simulink model "Three_phase_twelve_pulse_wave"  (R2025a)
settings: Solver=VariableStepAuto  StartTime=0.0  StopTime=0.06  MaxStep=1e-4  RelTol=1e-3
undefined symbols (not defined in the file): D1, Delta, lagging, pulse
libraries: spsUniversalBridgeLib x2, spsGroundLib x1, spsMultimeterLib x1, spsPLL3phLib x1, spsPulseGeneratorThyristor12PulseLib x1, spsSeriesRLCBranchLib x1, spsThreePhaseProgrammableVoltageSourceLib x1, spsThreePhaseVIMeasurementLib x1, spsThreePhaseTransformerThreeWindingsLib x1, sps_lib x1
settings Model: Creator=wz  LastModifiedBy=wz

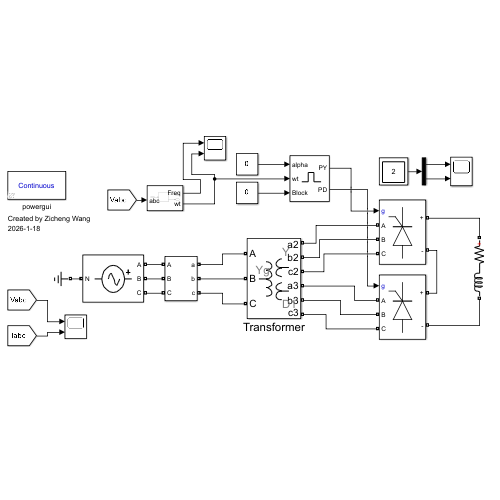
[thumbnail: Simulink's stored preview of the top-level diagram]
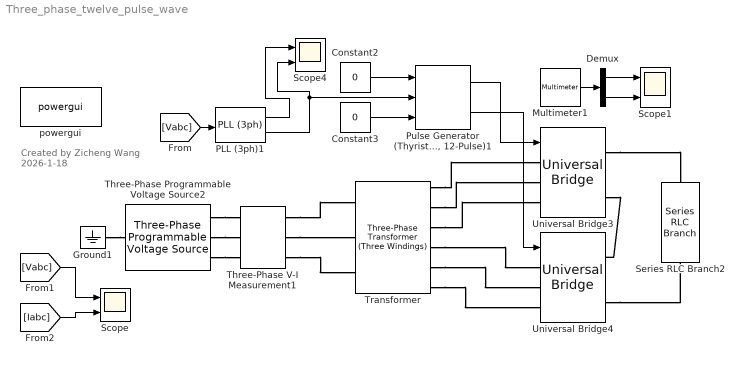
== system Three_phase_twelve_pulse_wave ==
  note: Created by Zicheng Wang
      | 2026-1-18
  Constant2 : Constant  Value=0
  Constant3 : Constant  Value=0
  Demux : Demux  Outputs=2
  Ground1 : spsGroundLib/Ground  LConnTagsString=a
  Multimeter1 : spsMultimeterLib/Multimeter  L=11  sel=[1 2]  yselected={}  Gain=[1 1]  OutputType=Complex  PlotAtSimulationStop=off  PhasorSimulation=off
  PLL (3ph)1 : spsPLL3phLib/PLL (3ph)  Fmin=49  Par_Init=[0, 50]  ParK=[180, 3200, 1]  TcD=1e-4  MaxRateChangeFreq=12  FilterCutOffFreq=25  Ts=0  AGC=on
  "Pulse Generator (Thyristor, 12-Pulse)1" : spsPulseGeneratorThyristor12PulseLib/Pulse Generator (Thyristor, 12-Pulse)  GenType=12-pulse  Delta=D1 (lagging)  pwidth=60  Double_Pulse=off  Ts=0
      settings: LibrarySourceBlock=|
      | sps_lib/Power Electronics/Power Electronics Control/Pulse Generator
      | (Thyristor, 12-Pulse)
  Scope : Scope  NumInputPorts=2
      settings: ActiveDisplayYMinimum=-387.83587594066989  ActiveDisplayYMaximum=387.83587594066989
  Scope1 : Scope  NumInputPorts=2
      settings: ActiveDisplayYMinimum=-129.6896842851543  ActiveDisplayYMaximum=1167.2071584549349
  Scope4 : Scope  NumInputPorts=2
      settings: ActiveDisplayYMinimum=-1  ActiveDisplayYMaximum=1  DataLoggingVariableName=ScopeData2
  Series RLC Branch2 : spsSeriesRLCBranchLib/Series RLC Branch  LConnTagsString=__new0  RConnTagsString=__new0  BranchType=RL  Resistance=10  Inductance=0.1  SetiL0=off  InitialCurrent=0  Capacitance=1e-6  Setx0=off  InitialVoltage=0  Measurements=Branch voltage and current
  Three-Phase Programmable Voltage Source2 : spsThreePhaseProgrammableVoltageSourceLib/Three-Phase Programmable Voltage Source  PositiveSequence="[380  0 50]"  VariationEntity=None  VariationType=Table of time-amplitude pairs  VariationTypeAlt=Step  VariationStep=0.5  VariationRate=10  VariationMagnitude=0.3  VariationFrequency=2  VariationTiming=[1 2]  VariationPhaseA=off  Amplitudes=[1 0.8 1.2 1.0]  TimeValues=[0 0.1 0.15 0.2]  HarmonicGeneration=off  HarmonicA=[3 0.2 -25 0]  HarmonicB=[2 0.15 35 2]  Timing="[0.05  3]"  BusType=swing  Pref=0  Qref=0  Qmin=-inf  Qmax=inf
  Three-Phase V-I Measurement1 : spsThreePhaseVIMeasurementLib/Three-Phase V-I Measurement  VoltageMeasurement=phase-to-ground  SetLabelV=on  LabelV=Vabc  Vpu=off  VpuLL=off  CurrentMeasurement=yes  SetLabelI=on  LabelI=Iabc  Ipu=off  Pbase=100e6  Vbase=500e3  OutputType=Complex  PhasorSimulation=off  PSBequivalent=0
  Transformer : spsThreePhaseTransformerThreeWindingsLib/Three-Phase Transformer (Three Windings)  Winding1Connection=Yg  Winding2Connection=Y  Winding3Connection=Delta (D1)  CoreType=Three single-phase transformers  SetSaturation=off  Hysteresis=off  DataFile='basic_model'  SetInitialFlux=off  Measurements=Winding currents  UNITS=pu  NominalPower=[ 1200e6 , 50 ]  Winding1="[ 200e3 0  0 ]"  Winding2=[ 200e3 0 0]  Winding3=[ 200e3 0.001 0]  Rm=500  Lm=500  L0=0.5  Saturation=[0 0; 1 1.2; 2 1.1]  InitialFluxes=[0.8 -0.8 0.7]  BreakLoop=off  DiscreteSolver=Trapezoidal iterative  DataType=off  TransfoNumber=0
      settings: AttributesFormatString=\n
  Universal Bridge3 : spsUniversalBridgeLib/Universal Bridge  Arms=3  SnubberResistance=1e5  SnubberCapacitance=inf  Device=Thyristors  Ron=1e-3  Lon=0  ForwardVoltages="[  0  0  ]"  ForwardVoltage=0  GTOparameters=[ 10e-6 , 20e-6 ]  IGBTparameters=[ 1e-6 , 2e-6 ]  Measurements=None  Measurements_2=None  converterType=Rectifier
  Universal Bridge4 : spsUniversalBridgeLib/Universal Bridge  Arms=3  SnubberResistance=1e5  SnubberCapacitance=inf  Device=Thyristors  Ron=1e-3  Lon=0  ForwardVoltages="[  0  0  ]"  ForwardVoltage=0  GTOparameters=[ 10e-6 , 20e-6 ]  IGBTparameters=[ 1e-6 , 2e-6 ]  Measurements=None  Measurements_2=None  converterType=Rectifier
  powergui : sps_lib/powergui  Priority=1  SimulationMode=Continuous  SampleTime=50e-6  frequency=60  Iterations=50  frequencyindice=50  Pbase=100e6  ErrMax=1e-4  UnitsV=kV  UnitsW=MW  buscounter=0  FunctionMessages=off  echomessages=off  EnableUseOfTLC=off  CurrentSourceSwitches=off  DisableSnubberDevices=off  DisableRonSwitches=off  DisableVfSwitches=off  DisplayEquations=off  AutomaticDiscreteSolvers=off  SolverType=Tustin/Backward Euler (TBE)  Interpol=off  ExternalGateDelay=off  methode=off  Ts=100  x0status=blocks  SPID=on  SwTol=0  HookPort=off  NonlinearTolerance=1e-4  nMaxIteration=100  ContinueOnMaxIteration=off  RestoreLinks=warning  ResistiveCurrentMeasurement=off  Frange=[0:2:500]  Ylog=off  Xlog=on  ShowGrid=off  save=off  variable=ZData  structure=0  ZoomFFT=off  StartTime=0.0  cycles=1  DisplayStyle=1  fundamental=60  FreqAxis=off  MaxFrequency=1000  frequencyindicesteady=1  RmsSteady=1  display=off
  wires:
  PLL (3ph)1/1 -> Scope4/1
  PLL (3ph)1/2 -> Scope4/2, "Pulse Generator (Thyristor, 12-Pulse)1"/2
  Constant2/1 -> "Pulse Generator (Thyristor, 12-Pulse)1"/1
  Constant3/1 -> "Pulse Generator (Thyristor, 12-Pulse)1"/3
  "Pulse Generator (Thyristor, 12-Pulse)1"/1 -> Universal Bridge3/1
  "Pulse Generator (Thyristor, 12-Pulse)1"/2 -> Universal Bridge4/1
  [Vabc] -> PLL (3ph)1/1
  [Vabc] -> Scope/1
  [Iabc] -> Scope/2
  Multimeter1/1 -> Demux/1
  Demux/1 -> Scope1/1
  Demux/2 -> Scope1/2
  connections:
  Three-Phase Programmable Voltage Source2/RConn3 -- Three-Phase V-I Measurement1/LConn3
  Three-Phase Programmable Voltage Source2/RConn2 -- Three-Phase V-I Measurement1/LConn2
  Ground1/LConn1 -- Three-Phase Programmable Voltage Source2/LConn1
  Three-Phase Programmable Voltage Source2/RConn1 -- Three-Phase V-I Measurement1/LConn1
  Universal Bridge4/RConn2 -- Series RLC Branch2/RConn1
  Universal Bridge3/RConn1 -- Series RLC Branch2/LConn1
  Universal Bridge3/RConn2 -- Universal Bridge4/RConn1
  Three-Phase V-I Measurement1/RConn1 -- Transformer/LConn1
  Three-Phase V-I Measurement1/RConn2 -- Transformer/LConn2
  Three-Phase V-I Measurement1/RConn3 -- Transformer/LConn3
  Transformer/RConn1 -- Universal Bridge3/LConn1
  Transformer/RConn2 -- Universal Bridge3/LConn2
  Transformer/RConn3 -- Universal Bridge3/LConn3
  Transformer/RConn4 -- Universal Bridge4/LConn1
  Transformer/RConn5 -- Universal Bridge4/LConn2
  Transformer/RConn6 -- Universal Bridge4/LConn3
